simulink model "p560Project_jacobian"  (R2020b)
settings: Solver=VariableStepAuto  StartTime=0.0  StopTime=16  RelTol=1e-3
undefined symbols (not defined in the file or in its folder): DiscIntNeverNeededParam, qn
libraries: roblocks x5, simulink x1
settings Model: Creator=Valentina  LastModifiedBy=Valentina

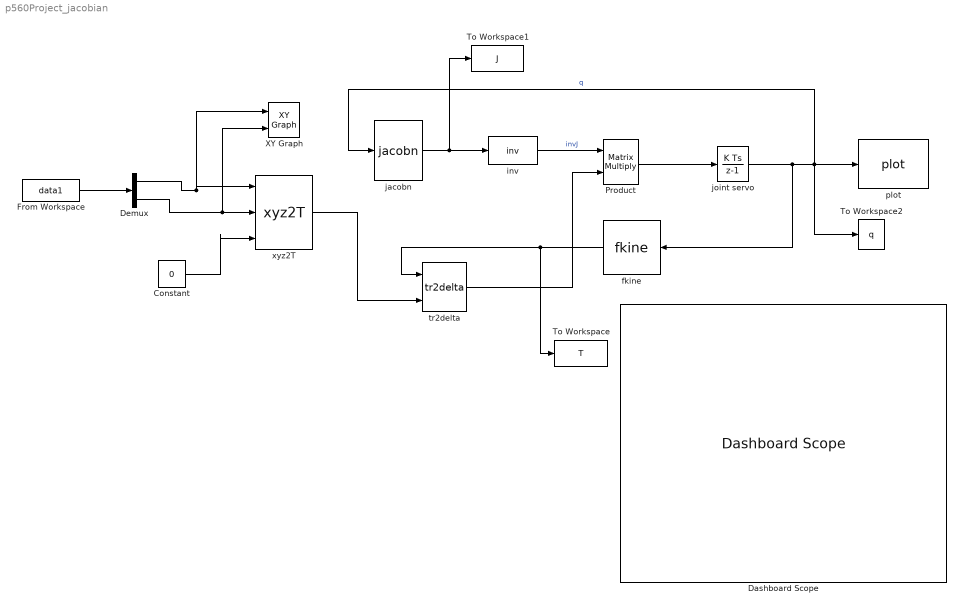
== system p560Project_jacobian ==
  Constant : Constant  Value=0
  Dashboard Scope : DashboardScope
  Demux : Demux  Outputs=2
  From Workspace : FromWorkspace  VariableName=data1  SampleTime=-1
  Product : Product  Multiplication=Matrix(*)  InputSameDT=on  RndMeth=Zero  SaturateOnIntegerOverflow=on  OutDataTypeStr=Inherit: Same as first input
  To Workspace : ToWorkspace  VariableName=T  SampleTime=-1
  To Workspace1 : ToWorkspace  VariableName=J  SampleTime=-1
  To Workspace2 : ToWorkspace  VariableName=q  SampleTime=-1
  XY Graph : simulink/Sinks/XY Graph  xmin=-1  xmax=1  ymin=-1  ymax=1  st=-1
  fkine : roblocks/Arm/fkine  robot=p560
  inv : MATLABFcn  MATLABFcn=inv  Output1D=off
  jacobn : roblocks/Arm/jacobn  robot=p560
  joint servo : DiscreteIntegrator  gainval=5  InitialCondition=qn  SampleTime=0.05  ICPrevOutput=DiscIntNeverNeededParam  ICPrevScaledInput=DiscIntNeverNeededParam
  plot : roblocks/Arm/plot  robot=p560  fps=5  holdplot=on
  tr2delta : roblocks/Toolbox/tr2delta
  xyz2T : roblocks/Toolbox/xyz2T
  wires:
  jacobn/1 -> inv/1, To Workspace1/1
  inv/1 -> Product/1  "invJ"
  Product/1 -> joint servo/1
  joint servo/1 -> fkine/1, jacobn/1, To Workspace2/1, plot/1  "q"
  xyz2T/1 -> tr2delta/2
  tr2delta/1 -> Product/2
  fkine/1 -> To Workspace/1, tr2delta/1
  Demux/2 -> XY Graph/2, xyz2T/2
  Demux/1 -> XY Graph/1, xyz2T/1
  From Workspace/1 -> Demux/1
  Constant/1 -> xyz2T/3
